simulink model "mirageTrackingRobot"  (R2015a)
settings: Solver=FixedStepDiscrete  StartTime=0.0  StopTime=10.0  FixedStep=0.2  RelTol=1e-3
undefined symbols (not defined in the file or in its folder): RGB24
libraries: xpcvideousblib x2, slrtlib x1
settings Model: Creator=sd0016  LastModifiedBy=sd0016
settings SolverCC: EnableConcurrentExecution=on
settings OptimizationCC: BlockReduction=off  OptimizeBlockIOStorage=off  BufferReuse=off  GlobalBufferReuse=off  ExpressionFolding=off  LocalBlockOutputs=off
settings HardwareCC: ProdIntDivRoundTo=Zero  ProdEndianess=LittleEndian  ProdLongLongMode=on  ProdHWDeviceType=Generic->32-bit x86 compatible
settings RTWCC: SystemTargetFile=slrt.tlc  TemplateMakefile=slrt_default_tmf  Description=Simulink Real-Time  RTWCompilerOptimization=on
settings SimulinkRealTimeCC: GeneratePreprocessorConditionals=Disable all

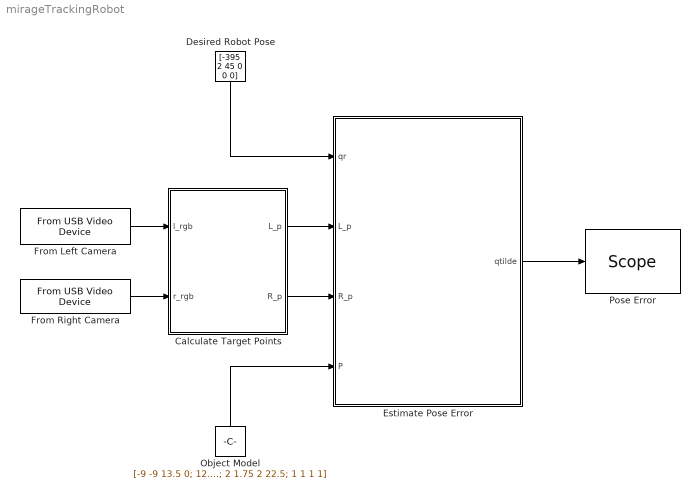
== system mirageTrackingRobot ==
  Calculate Target Points : MATLAB Function  TreatAsAtomicUnit=on
  Desired Robot Pose : Constant  Value=[-395 2 45 0 0 0]
  Estimate Pose Error : MATLAB Function  TreatAsAtomicUnit=on
  From Left Camera : xpcvideousblib/From USB Video Device  sconf=<Select a configuration>  paddr=-1  iwidth=1280  iheight=960  fint=1/5  ffmt=Uncompressed  cfmt=RGB24 (8:8:8)  isig=One multidimensional signal  trigger=off  status=off  updateBlock=1
  From Right Camera : xpcvideousblib/From USB Video Device  sconf=<Select a configuration>  paddr=-1  iwidth=1280  iheight=960  fint=1/5  ffmt=Uncompressed  cfmt=RGB24 (8:8:8)  isig=One multidimensional signal  trigger=off  status=off  updateBlock=1
  Object Model : Constant  Value=[-9 -9 13.5 0; 12.75 -12.75 0 0; 2 1.75 2 22.5; 1 1 1 1]
  "Pose Error " : slrtlib/Displays and Logging/Scope   scopeno=1  scopetype=Target  autostart=on  viewmode=Graphical redraw  formatstr='%15.6f'  grid=on  ylimits=[0,0]  nosamples=3  noprepostsamples=0  interleave=1  triggermode=FreeRun  triggersignal=1  trigsignalfromport=off  triggerlevel=0.0  triggerslope=Either  triggerscope=1  triggersample=0  filename=data.dat  mode=Lazy  writesize=512  autorestart=off  dynamicfilemode=off  maxwritefilesize=512*1024^2
  wires:
  From Right Camera/1 -> Calculate Target Points/2(r_rgb)
  From Left Camera/1 -> Calculate Target Points/1(l_rgb)
  Calculate Target Points/1(L_p) -> Estimate Pose Error/2(L_p)
  Calculate Target Points/2(R_p) -> Estimate Pose Error/3(R_p)
  Desired Robot Pose/1 -> Estimate Pose Error/1(qr)
  Object Model/1 -> Estimate Pose Error/4(P)
  Estimate Pose Error/1(qtilde) -> "Pose Error "/1

== matlab function mirageTrackingRobot/Calculate Target Points ==
  data: l_rgb input; L_p output; r_rgb input; R_p output
function [L_p, R_p] = getCenter(l_rgb,r_rgb)

    %#codegen
    L_p=zeros(2,4);
    R_p=zeros(2,4);
    
    %input left image(l_rgb), right image(r_rgb), Pose target position 
    [m,n,c]=size(l_rgb);
    
    %define image variables for processing
    l_gray=zeros(m,n);      r_gray=zeros(m,n);
    l_rgb1=zeros(m,n,c);    r_rgb1=zeros(m,n,c);
    l_rgb2=zeros(m,n);      r_rgb2=zeros(m,n);

    l_bw=false(m,n);        r_bw=false(m,n);

    l_rgb1 = imcomplement(l_rgb);        % converts RGB to CMY color space 
    r_rgb1 = imcomplement(r_rgb);        % converts RGB to CMY color space 
    
    l_gray = 0.2989 * l_rgb1(:,:,1) + 0.5870 * l_rgb1(:,:,2) + 0.1140 * l_rgb1(:,:,3); % rgb2gray(rgb) ;convert rgb to grayscale 
    r_gray = 0.2989 * r_rgb1(:,:,1) + 0.5870 * r_rgb1(:,:,2) + 0.1140 * r_rgb1(:,:,3); % rgb2gray(rgb) ;convert rgb to grayscale
    
    l_rgb2 = l_rgb1(:,:,3)-l_gray;       % imsubtract(rgb1(:,:,3),gray)
    r_rgb2 = r_rgb1(:,:,3)-r_gray;       % imsubtract(rgb1(:,:,3),gray) 
    
    l_rgb2 = medfilt2(l_rgb2);     % medfilt2(rgb2,[3 3]);
    r_rgb2 = medfilt2(r_rgb2);     % medfilt2(rgb2,[3 3]);
    
    l_rgb2 = myMat2gray(l_rgb2);
    r_rgb2 = myMat2gray(r_rgb2);
    
    l_bw = l_rgb2 > 0.6;
    r_bw = r_rgb2 > 0.6;

    %finds yellow regions in image using BlobAnalysis.
    hblob = vision.BlobAnalysis;

    [~,l_center,~] = step(hblob, l_bw); % get [x y] is a centroid of region
    [~,r_center,~] = step(hblob, r_bw); % get [x y] is a centroid of region
    
    %Send Left Camera Points
    ml = size(l_center,1);
    if ml > 4
        ml = 4;
    end
    for i=1:ml
        L_p(:,i)=l_center(i,:);
    end
    
    %Send Right Camera Points
    mr = size(r_center,1);
    if mr > 4
        mr = 4;
    end
    for i=1:mr
        R_p(:,i)=r_center(i,:);
    end
    
    L_p = orderPoints(L_p); 
    R_p = orderPoints(R_p);
    
%     coder.extrinsic('imshow','plot');
%     imshow(l_rgb2);hold on;
%     plot(L_p(1,:),L_p(2,:),'ro');
    
    L_p(2,:) = m - L_p(2,:);
    R_p(2,:) = m - R_p(2,:);
end

function imgOut = myMat2gray(imgIn)
    %#codegen
    imgIn = double(imgIn);
    
    minL = min(imgIn(:));
    
    imgTmp = (imgIn - minL);
    
    maxL = max(imgTmp(:));
    
    imgOut = imgTmp/maxL;
end

== matlab function mirageTrackingRobot/Estimate Pose Error ==
  data: qr input; qtilde output; L_p input; R_p input; P input
function qtilde = mirage(qr,L_p,R_p,P)
%#codegen

%Desired Robot Pose for current step qr()
robotPoseDes.x = qr(1);
robotPoseDes.y = qr(2);
robotPoseDes.z = qr(3);
robotPoseDes.phi = qr(4);
robotPoseDes.theta = qr(5);
robotPoseDes.psi = qr(6);

%Transform target points from I space into Desired Robot Space
world2robotDes = inv(EulerTrans(robotPoseDes));
S_PDes = world2robotDes*P;

%Calculate the error parameters for current step
errParams = visioMotor(L_p,R_p,S_PDes);

poseErrorMat = eye(4,4);
poseErrorMat(1:3,:) = reshape(errParams,3,4);

world2robot = poseErrorMat*world2robotDes;

robotPoseEst = calculatePose(world2robot);

qtilde = [ -robotPoseEst.x  - robotPoseDes.x;
           -robotPoseEst.y  - robotPoseDes.y;
           -robotPoseEst.z  - robotPoseDes.z;
           -robotPoseEst.phi  - robotPoseDes.phi;
           -robotPoseEst.theta  - robotPoseDes.theta;
           -robotPoseEst.psi  - robotPoseDes.psi;];
       
end
